simulink model "costas_loop_V2"  (R2013b)
settings: Solver=ode3  StartTime=0.0  StopTime=10e3/1200  FixedStep=1/480e3  RelTol=1e-3
libraries: dsparch4 x3, commsynccomp2 x2, commrandsrc2 x1, commchan3 x1, commsink2 x1, commfilt2 x1
settings Model: Creator=tibbs2010  LastModifiedBy=owner
settings DebuggingCC: StateNameClashWarn=warning

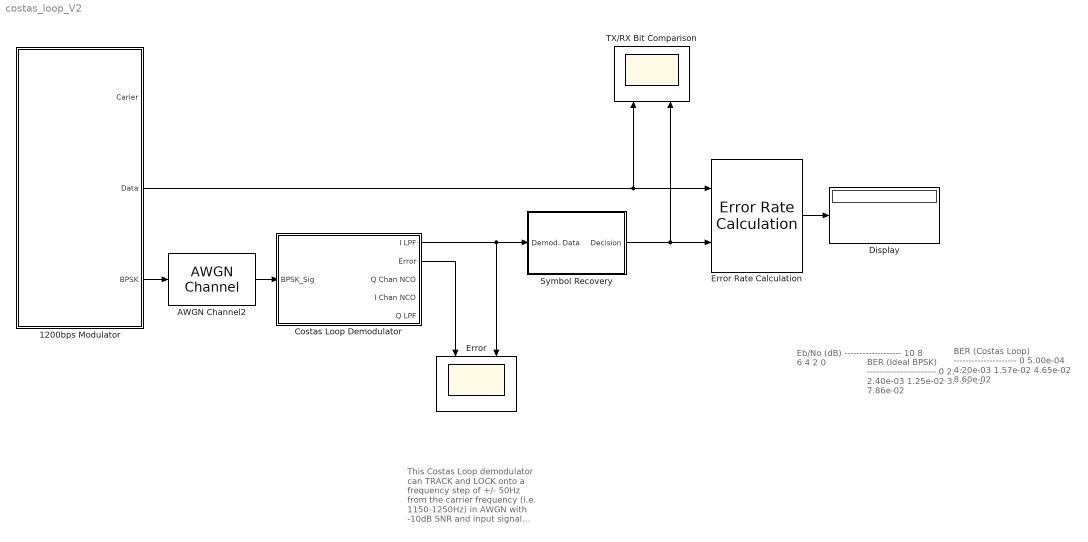
== system costas_loop_V2 ==
  note: This Costas Loop demodulator can TRACK and LOCK onto a
      |  frequency step of +/- 50Hz from the carrier frequency (i.e. 1150-1250Hz)
      | in AWGN with -10dB SNR and input signal power of 0.5W.
  note: BER (Ideal BPSK)
      | -----------------------
      | 0
      | 2.00e-04
      | 2.40e-03
      | 1.25e-02
      | 3.75e-02
      | 7.86e-02
  note: Eb/No (dB)
      | -------------------
      | 10
      | 8
      | 6
      | 4
      | 2
      | 0
  note: BER (Costas Loop)
      | ---------------------
      | 0
      | 5.00e-04
      | 4.20e-03
      | 1.57e-02
      | 4.65e-02
      | 8.60e-02
  1200bps Modulator : Subsystem
  AWGN Channel2 : commchan3/AWGN Channel  InputProcessing=Columns as channels (frame based)  seed=randseed  noiseMode="Signal to noise ratio  (Eb/No)"  EbNodB=0  EsNodB=10  SNRdB=10  bitsPerSym=1  Ps=12.5  Tsym=1/1200  variance=1
  Costas Loop Demodulator : Subsystem
  Display : Display
  Error : Scope  NumInputPorts=2
      settings: YMin=-0.9~-2  YMax=0.7~2  SaveName=ScopeData2
  Error Rate Calculation : commsink2/Error Rate Calculation  N=1  st_delay=0  cp_mode=Entire frame  subframe=[]  PMode=Port  WsName=ErrorVec  RsMode2=off  stop=off  numErr=100  maxBits=1e6
  Symbol Recovery : Subsystem
  TX/RX Bit Comparison : Scope  NumInputPorts=2
      settings: YMin=-0.3~-2  YMax=2~2
  wires:
  Costas Loop Demodulator/1(I LPF) -> Symbol Recovery/1(Demod. Data), Error/2
  Symbol Recovery/1(Decision) -> Error Rate Calculation/2, TX/RX Bit Comparison/2
  Error Rate Calculation/1 -> Display/1
  Costas Loop Demodulator/2(Error) -> Error/1
  1200bps Modulator/3(BPSK) -> AWGN Channel2/1
  AWGN Channel2/1 -> Costas Loop Demodulator/1(BPSK_Sig)
  1200bps Modulator/2(Data) -> TX/RX Bit Comparison/1, Error Rate Calculation/1

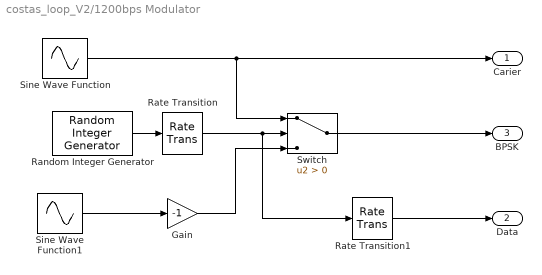
== system costas_loop_V2/1200bps Modulator ==
  Gain : Gain  Gain=-1
  Random Integer Generator : commrandsrc2/Random Integer Generator  mul=2  seed=randseed  Ts=1/1200  frameBased=off  sampPerFrame=1  orient=off  outDataType=double
  Rate Transition : RateTransition  OutPortSampleTime=1/480e3
  Rate Transition1 : RateTransition  OutPortSampleTime=1/1200
  Sine Wave Function : Sin  Amplitude=5  Frequency=2*pi*2400  Phase=pi/2  SampleTime=1/480e3
  Sine Wave Function1 : Sin  Amplitude=5  Frequency=2*pi*2400  Phase=pi/2  SampleTime=1/480e3
  Switch : Switch  Criteria=u2 > Threshold
  Carier : Outport
  Data : Outport  Port=2
  BPSK : Outport  Port=3
  wires:
  Random Integer Generator/1 -> Rate Transition/1
  Rate Transition/1 -> Rate Transition1/1, Switch/2
  Sine Wave Function/1 -> Carier/1, Switch/1
  Sine Wave Function1/1 -> Gain/1
  Gain/1 -> Switch/3
  Switch/1 -> BPSK/1
  Rate Transition1/1 -> Data/1

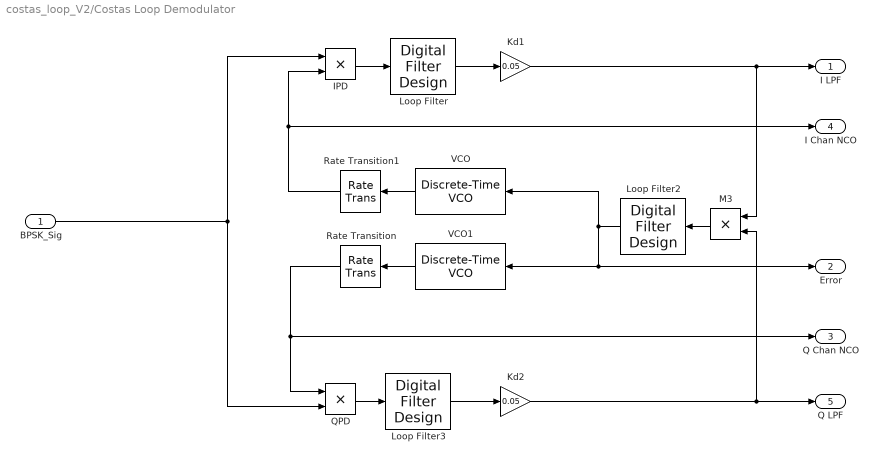
== system costas_loop_V2/Costas Loop Demodulator ==
  BPSK_Sig : Inport
  IPD : Product
  Kd1 : Gain  Gain=0.05
  Kd2 : Gain  Gain=0.05
  Loop Filter : dsparch4/Digital Filter Design  mwdsp_browser_bugfix_var=off
  Loop Filter2 : dsparch4/Digital Filter Design  mwdsp_browser_bugfix_var=off
  Loop Filter3 : dsparch4/Digital Filter Design  mwdsp_browser_bugfix_var=off
  M3 : Product
  QPD : Product
  Rate Transition : RateTransition  OutPortSampleTime=1/480e3
  Rate Transition1 : RateTransition  OutPortSampleTime=1/480e3
  VCO : commsynccomp2/Discrete-Time VCO  Ac=5  Fc=2400  Kc=.5  Ph=0  ts=1/480e3
  VCO1 : commsynccomp2/Discrete-Time VCO  Ac=5  Fc=2400  Kc=.5  Ph=pi/2  ts=1/480e3
  I LPF : Outport
  Error : Outport  Port=2
  Q Chan NCO : Outport  Port=3
  I Chan NCO : Outport  Port=4
  Q LPF : Outport  Port=5
  wires:
  VCO/1 -> Rate Transition1/1
  VCO1/1 -> Rate Transition/1
  Loop Filter3/1 -> Kd2/1
  QPD/1 -> Loop Filter3/1
  Rate Transition/1 -> QPD/1, Q Chan NCO/1
  Rate Transition1/1 -> IPD/2, I Chan NCO/1
  IPD/1 -> Loop Filter/1
  Loop Filter/1 -> Kd1/1
  M3/1 -> Loop Filter2/1
  Loop Filter2/1 -> VCO/1, Error/1, VCO1/1
  Kd2/1 -> Q LPF/1, M3/2
  Kd1/1 -> I LPF/1, M3/1
  BPSK_Sig/1 -> IPD/1, QPD/2

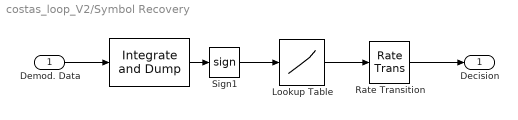
== system costas_loop_V2/Symbol Recovery ==
  Demod. Data : Inport
  " " : commfilt2/Integrate and Dump  obssamples=400  offsetsamples=0  nodump=off  roundingMode=Floor  overflowMode=off
  Lookup Table : Lookup  InputValues=[-1,0,1]  Table=[0,0,1]
  Rate Transition : RateTransition  OutPortSampleTime=1/1200
  Sign1 : Signum
  Decision : Outport
  wires:
  Demod. Data/1 -> " "/1
  Sign1/1 -> Lookup Table/1
  Rate Transition/1 -> Decision/1
  " "/1 -> Sign1/1
  Lookup Table/1 -> Rate Transition/1
